simulink model "controller"  (R2024a)
settings: Solver=FixedStepAuto  StartTime=0.0  StopTime=10.0  FixedStep=1/100  RelTol=1e-3
undefined symbols (not defined in the file): MAX_TORQUE, MAX_TORQUE_REVERSE, TransmissionState
settings Model: Creator=DAUIN-Win10  LastModifiedBy=lucap
settings OptimizationCC: ReuseModelBlockBuffer=off
settings DebuggingCC: UnconnectedInputMsg=warning  UnconnectedOutputMsg=warning  UnconnectedLineMsg=warning
settings ModelReferenceCC: EnableRefExpFcnMdlSchedulingChecks=on
settings RTWCC: GPUComputeCapability=3.5  DLArmComputeVersion=19.05

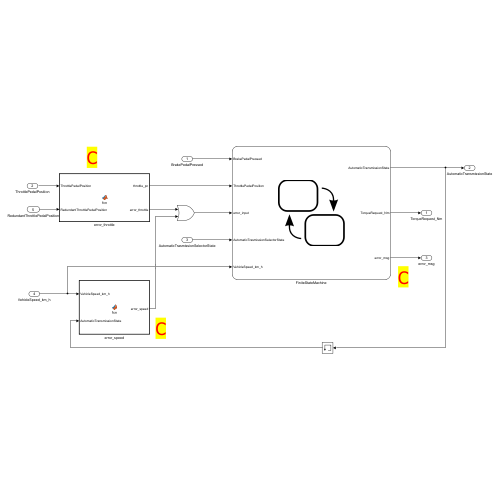
[thumbnail: Simulink's stored preview of the top-level diagram]
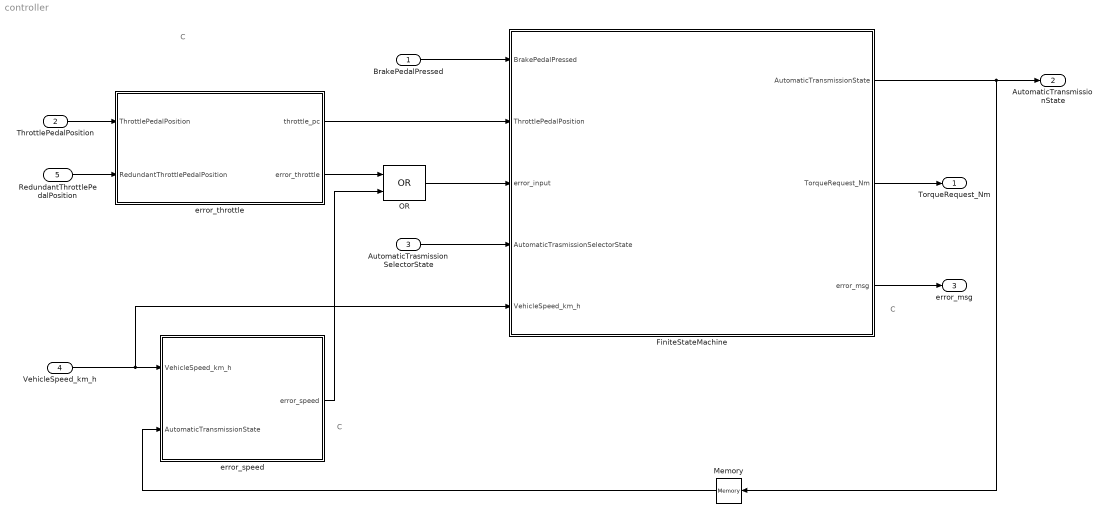
== system controller ==
  note: C
  note: C
  note: C
  BrakePedalPressed : Inport  OutDataTypeStr=boolean
  ThrottlePedalPosition : Inport  Port=2  OutDataTypeStr=single
  AutomaticTrasmissionSelectorState : Inport  Port=3  OutDataTypeStr=Enum: TransmissionState
  VehicleSpeed_km_h : Inport  Port=4  OutDataTypeStr=single  Unit=km/h
  RedundantThrottlePedalPosition : Inport  Port=5  OutDataTypeStr=single
  FiniteStateMachine : Stateflow chart  TreatAsAtomicUnit=on
      settings: PortSchema="{\"entries\":[{\"content\":{\"sides\":[{\"content\":{\"connectorIds\":[\"In1\",\"In2\",\"In5\",\"In3\",\"In4\"]},\"type\":\"ConnectorPlacement.EquallySpacedRectSide\",\"uuid\":\"bf31f6ae-db8c-4ab1-ad77-5a3ef50bcb9a\"},{\"content\":{\"connectorIds\":[\"Out1\",\"Out2\",\"Out3\"],\"side\":\"RIGHT\"},\"type\":\"ConnectorPlacement.EquallySpacedRectSide\",\"uuid\":\"4709d2a0-a250-4961-944b-22e44bd393fa\"},{\"content\":{\"side\":\"TOP\"},\"type\":\"ConnectorPlacement.EquallySpacedRectSide\",\"uuid\":\"e821ed33-8c78-4d62-9a28-a1088cc256b0\"}]},\"type\":\"ConnectorPlacement.EquallySpacedConnector\",\"uuid\":\"de898920-7aae-487c-983f-219140b217f5\"}],\"packageUris\":[\"http://schema.mathworks.com/mf0/Connector/R2020b\"],\"version\":\"1.0\"}"
  Memory : Memory  InitialCondition=TransmissionState.Park
  OR : Logic  Operator=OR  IconShape=distinctive  AllPortsSameDT=off  OutDataTypeStr=boolean
  error_speed : MATLAB Function  TreatAsAtomicUnit=on
  error_throttle : MATLAB Function  TreatAsAtomicUnit=on
  TorqueRequest_Nm : Outport  OutDataTypeStr=single  Unit=N*m
  AutomaticTransmissionState : Outport  Port=2  OutDataTypeStr=Enum: TransmissionState
  error_msg : Outport  Port=3  OutDataTypeStr=boolean  Unit=N*m
  wires:
  BrakePedalPressed/1 -> FiniteStateMachine/1(BrakePedalPressed)
  ThrottlePedalPosition/1 -> error_throttle/1(ThrottlePedalPosition)
  AutomaticTrasmissionSelectorState/1 -> FiniteStateMachine/3(AutomaticTrasmissionSelectorState)
  FiniteStateMachine/1(AutomaticTransmissionState) -> AutomaticTransmissionState/1, Memory/1
  FiniteStateMachine/2(TorqueRequest_Nm) -> TorqueRequest_Nm/1
  RedundantThrottlePedalPosition/1 -> error_throttle/2(RedundantThrottlePedalPosition)
  FiniteStateMachine/3(error_msg) -> error_msg/1
  error_throttle/1(throttle_pc) -> FiniteStateMachine/2(ThrottlePedalPosition)
  VehicleSpeed_km_h/1 -> FiniteStateMachine/4(VehicleSpeed_km_h), error_speed/1(VehicleSpeed_km_h)
  error_throttle/2(error_throttle) -> OR/1
  error_speed/1(error_speed) -> OR/2
  OR/1 -> FiniteStateMachine/5(error_input)
  Memory/1 -> error_speed/2(AutomaticTransmissionState)

== matlab function controller/error_throttle ==
  data: throttle_pc output; ThrottlePedalPosition input; error_throttle output; RedundantThrottlePedalPosition input
function [throttle_pc, error_throttle]  = fcn(ThrottlePedalPosition, RedundantThrottlePedalPosition)

diff = abs(ThrottlePedalPosition - RedundantThrottlePedalPosition);
diff = round(diff * 1000) / 1000; % avoid matlab numerical errors

if diff > 0.05
    error_throttle = boolean(1);
    throttle_pc = single(-1);
else
    error_throttle = boolean(0);
    throttle_pc = single(ThrottlePedalPosition);
end

== stateflow chart controller/FiniteStateMachine ==
  state Init
  state correctly_working
    state P
      entry:
      AutomaticTransmissionState = TransmissionState.Park
      TorqueRequest_Nm = 0
    state B
      entry:
      AutomaticTransmissionState = TransmissionState.Brake;
      state B_acc
        during:
        TorqueRequest_Nm = MAX_TORQUE * (3/2) * (ThrottlePedalPosition - 1/3)
      state B_dec
        during:
        TorqueRequest_Nm = -MAX_TORQUE * (1 - 3*ThrottlePedalPosition)
      state B_do_nothing
        entry:
        TorqueRequest_Nm = 0;
      B_acc -> B_dec : [ThrottlePedalPosition > 0 && ThrottlePedalPosition <= 1/3]
      B_dec -> B_acc [order 1] : [ThrottlePedalPosition > 1/3 && ThrottlePedalPosition <= 1]
      B_do_nothing -> B_acc : [ThrottlePedalPosition > 1/3 && ThrottlePedalPosition <= 1]
      B_dec -> B_do_nothing [order 2] : [VehicleSpeed_km_h <= 0]
      (default) -> B_do_nothing
    state D
      entry:
      AutomaticTransmissionState = TransmissionState.Drive
      during:
      TorqueRequest_Nm = MAX_TORQUE * ThrottlePedalPosition
    state N
      entry:
      AutomaticTransmissionState = TransmissionState.Neutral
      TorqueRequest_Nm = 0
    state R
      entry:
      AutomaticTransmissionState = TransmissionState.Reverse
      during:
      TorqueRequest_Nm = -MAX_TORQUE_REVERSE * ThrottlePedalPosition
    P -> B [order 2] : [ AutomaticTrasmissionSelectorState == TransmissionState.Brake && BrakePedalPressed == 1 && VehicleSpeed_km_h > -5]
    (default) -> P
    N -> P [order 2] : [abs(VehicleSpeed_km_h)<5 && BrakePedalPressed == 1 && AutomaticTrasmissionSelectorState == TransmissionState.Park]
    P -> N [order 1] : [AutomaticTrasmissionSelectorState == TransmissionState.Neutral && BrakePedalPressed == 1]
    B -> D : [AutomaticTrasmissionSelectorState == TransmissionState.Drive]
    D -> N [order 2] : [AutomaticTrasmissionSelectorState == TransmissionState.Neutral]
    N -> D [order 1] : [AutomaticTrasmissionSelectorState == TransmissionState.Drive && VehicleSpeed_km_h > -5 && BrakePedalPressed == 1]
    N -> R [order 3] : [VehicleSpeed_km_h < 5 && BrakePedalPressed == 1 && AutomaticTrasmissionSelectorState == TransmissionState.Reverse]
    D -> B [order 1] : [AutomaticTrasmissionSelectorState == TransmissionState.Brake]
    R -> N : [AutomaticTrasmissionSelectorState == TransmissionState.Neutral]
  state Error
    error_msg = boolean(1)
    TorqueRequest_Nm = 0
  (default) -> Init
  Init -> correctly_working : [error_input == 0 && ThrottlePedalPosition >= 0 && ThrottlePedalPosition <= 1]
  correctly_working -> Error : [error_input == 1]
  data: BrakePedalPressed input; ThrottlePedalPosition input single; AutomaticTrasmissionSelectorState input; VehicleSpeed_km_h input; AutomaticTransmissionState output; TorqueRequest_Nm output single; MAX_TORQUE parameter; MAX_TORQUE_REVERSE parameter; error_input input boolean =0; error_msg output

== matlab function controller/error_speed ==
  data: VehicleSpeed_km_h input; AutomaticTransmissionState input; error_speed output
function error_speed = fcn(VehicleSpeed_km_h, AutomaticTransmissionState)

if AutomaticTransmissionState == TransmissionState.Reverse && VehicleSpeed_km_h >= 5
        error_speed = boolean(1);
elseif AutomaticTransmissionState == TransmissionState.Park && abs(VehicleSpeed_km_h) >= 5
        error_speed = boolean(1);
elseif AutomaticTransmissionState == TransmissionState.Drive && VehicleSpeed_km_h <= -5
        error_speed = boolean(1);
elseif AutomaticTransmissionState == TransmissionState.Brake && VehicleSpeed_km_h <= -5
        error_speed = boolean(1);
else
    error_speed = boolean(0);
end
